simulink model "BicycleModelSimulink"  (R2017b)
settings: Solver=VariableStepAuto  StartTime=0.0  StopTime=0.4  FixedStep=0.001  MaxStep=0.010  MinStep=0.005  RelTol=1e-3  EnableMultiTasking=on
undefined symbols (not defined in the file): a, b, C_f, C_r, I_zz, m, step_steer
settings Model: Creator=tonylu  LastModifiedBy=tonylu
settings OptimizationCC: LifeSpan=inf
settings DebuggingCC: SFUnexpectedBacktrackingDiag=warning  SFNoUnconditionalDefaultTransitionDiag=warning  SFExecutionAtInitializationDiag=none
settings CodeAppCC: StateflowObjectComments=on
settings GRTTargetCC: TargetLangStandard=C89/C90 (ANSI)  GeneratePreprocessorConditionals=Disable all
settings ConfigComp: CovMetricSettings=dw  CovHtmlReporting=on  CovSaveCumulativeToWorkspaceVar=on  CovSaveSingleToWorkspaceVar=on  CovExternalEMLEnable=off

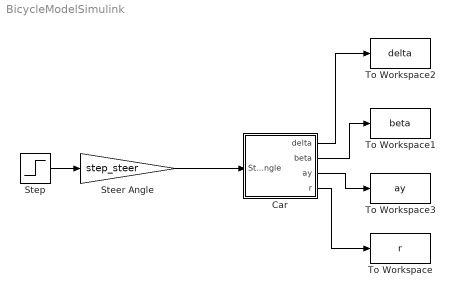
== system BicycleModelSimulink ==
  Car : Subsystem
  Steer Angle : Gain  Gain=step_steer
  Step : Step  Time=0  SampleTime=0
  To Workspace : ToWorkspace  VariableName=r  SaveFormat=Structure With Time  SampleTime=0.01
  To Workspace1 : ToWorkspace  VariableName=beta  SaveFormat=Structure With Time  SampleTime=0.01
  To Workspace2 : ToWorkspace  VariableName=delta  SaveFormat=Structure With Time  SampleTime=0.01
  To Workspace3 : ToWorkspace  VariableName=ay  SaveFormat=Structure With Time  SampleTime=0.01
  wires:
  Step/1 -> Steer Angle/1
  Car/1(delta) -> To Workspace2/1
  Car/2(beta) -> To Workspace1/1
  Car/3(ay) -> To Workspace3/1
  Car/4(r) -> To Workspace/1
  Steer Angle/1 -> Car/1(Steer Angle)

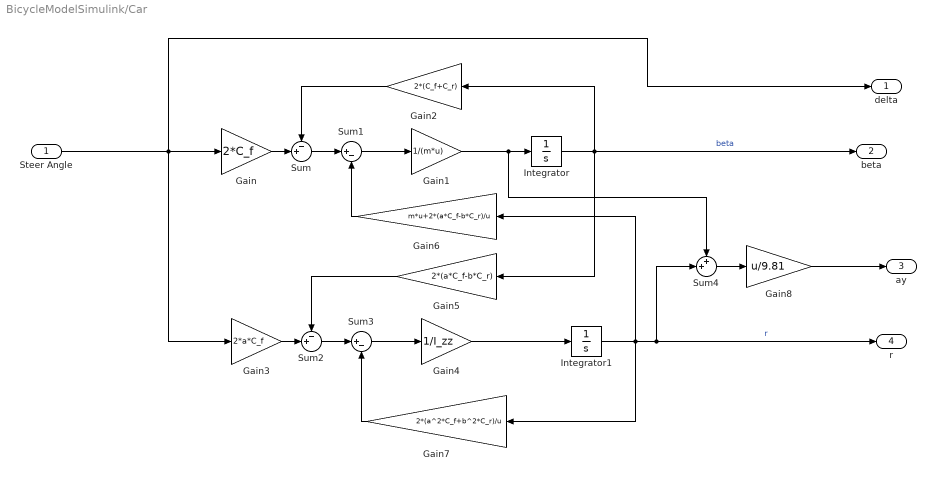
== system BicycleModelSimulink/Car ==
  Steer Angle : Inport
  Gain : Gain  Gain=2*C_f
  Gain1 : Gain  Gain=1/(m*u)
  Gain2 : Gain  Gain=2*(C_f+C_r)
  Gain3 : Gain  Gain=2*a*C_f
  Gain4 : Gain  Gain=1/I_zz
  Gain5 : Gain  Gain=2*(a*C_f-b*C_r)
  Gain6 : Gain  Gain=m*u+2*(a*C_f-b*C_r)/u
  Gain7 : Gain  Gain=2*(a^2*C_f+b^2*C_r)/u
  Gain8 : Gain  Gain=u/9.81
  Integrator : Integrator
  Integrator1 : Integrator
  Sum : Sum  Inputs=-+|
  Sum1 : Sum  Inputs=|+-
  Sum2 : Sum  Inputs=-+|
  Sum3 : Sum  Inputs=|+-
  Sum4 : Sum  Inputs=++|
  delta : Outport
  beta : Outport  Port=2
  ay : Outport  Port=3
  r : Outport  Port=4
  wires:
  Gain7/1 -> Sum3/2
  Sum4/1 -> Gain8/1
  Steer Angle/1 -> delta/1, Gain3/1, Gain/1
  Integrator/1 -> beta/1, Gain2/1, Gain5/1  "beta"
  Gain/1 -> Sum/2
  Gain4/1 -> Integrator1/1
  Gain1/1 -> Sum4/1, Integrator/1
  Gain2/1 -> Sum/1
  Sum2/1 -> Sum3/1
  Sum/1 -> Sum1/1
  Integrator1/1 -> r/1, Sum4/2, Gain7/1, Gain6/1  "r"
  Gain6/1 -> Sum1/2
  Gain3/1 -> Sum2/2
  Sum1/1 -> Gain1/1
  Gain5/1 -> Sum2/1
  Sum3/1 -> Gain4/1
  Gain8/1 -> ay/1
